simulink model "8Bit_Processor"  (R2019b)
settings: Solver=FixedStepDiscrete  StartTime=0.0  StopTime=10.0  RelTol=1e-3
libraries: hdlsllib x127, simulink_extras x9
(part 1 of 4)
settings Model: Creator=cohen  LastModifiedBy=cohen

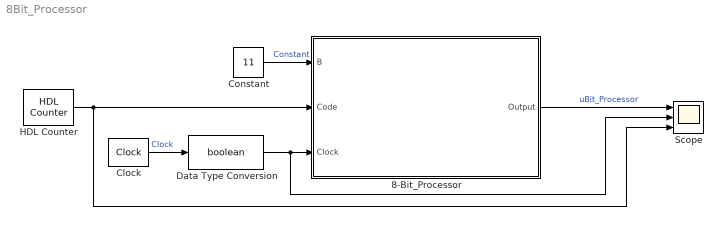
== system 8Bit_Processor ==
  8-Bit_Processor : Subsystem
  Clock : simulink_extras/Flip Flops/Clock  period=1
  Constant : Constant  Value=11  OutDataTypeStr=uint8  SampleTime=1
  Data Type Conversion : DataTypeConversion  OutDataTypeStr=boolean
  HDL Counter : hdlsllib/Sources/HDL Counter  CountType=Free running  CountInit=0  CountStep=1  CountMax=25  CountFromType=Initial value  CountFrom=0  CountResetPort=off  CountLoadPort=off  CountEnbPort=off  CountDirPort=off  CountDataType=Unsigned  CountWordLen=2  CountFracLen=0  CountSampTime=1
      settings: SourceProductName=Simulink
  Scope : Scope  NumInputPorts=3
  wires:
  Constant/1 -> 8-Bit_Processor/1(B)  "Constant"
  Clock/1 -> Data Type Conversion/1  "Clock"
  Data Type Conversion/1 -> Scope/2, 8-Bit_Processor/3(Clock)
  HDL Counter/1 -> Scope/3, 8-Bit_Processor/2(Code)
  8-Bit_Processor/1(Output) -> Scope/1  "uBit_Processor"

== system 8Bit_Processor/8-Bit_Processor ==
  B : Inport  OutDataTypeStr=uint8
  Code : Inport  Port=2
  Clock : Inport  Port=3
  8-Bit 4-to-1 MUX : Subsystem
  8-Bit_Adder : Subsystem
  8-Bit_Bitwise_AND : Subsystem
  8-Bit_Multiplier : Subsystem
  8-Bit_Register : Subsystem
  8-Bit_Subtractor : Subsystem
  Display : Display
  Display1 : Display
  Output : Outport  OutDataTypeStr=uint8
  wires:
  Code/1 -> 8-Bit 4-to-1 MUX/5(S)
  8-Bit 4-to-1 MUX/1(Out1) -> Output/1, Display/1, 8-Bit_Register/1(Data_In)
  Clock/1 -> 8-Bit_Register/2(Clk)
  8-Bit_Multiplier/1(Product) -> 8-Bit 4-to-1 MUX/2(In2)
  8-Bit_Bitwise_AND/1(Y) -> 8-Bit 4-to-1 MUX/4(In4)
  B/1 -> 8-Bit_Multiplier/2(B), 8-Bit_Subtractor/2(B), 8-Bit_Bitwise_AND/2(B), 8-Bit_Adder/2(B)
  8-Bit_Adder/1(Sum) -> 8-Bit 4-to-1 MUX/1(In1)
  8-Bit_Register/1(Data_out) -> Display1/1, 8-Bit_Adder/1(A), 8-Bit_Multiplier/1(A), 8-Bit_Subtractor/1(A), 8-Bit_Bitwise_AND/1(A)
  8-Bit_Subtractor/1(Difference) -> 8-Bit 4-to-1 MUX/3(In3)

== system 8Bit_Processor/8-Bit_Processor/8-Bit 4-to-1 MUX ==
  In1 : Inport  OutDataTypeStr=uint8
  In2 : Inport  Port=2  OutDataTypeStr=uint8
  In3 : Inport  Port=3  OutDataTypeStr=uint8
  In4 : Inport  Port=4  OutDataTypeStr=uint8
  S : Inport  Port=5
  Concat : Subsystem
  Slicer : Subsystem
  Slicer1 : Subsystem
  Slicer2 : Subsystem
  Slicer3 : Subsystem
  Subsystem : Subsystem
  Subsystem1 : Subsystem
  Subsystem2 : Subsystem
  Subsystem3 : Subsystem
  Subsystem4 : Subsystem
  Subsystem5 : Subsystem
  Subsystem6 : Subsystem
  Subsystem7 : Subsystem
  Out1 : Outport  OutDataTypeStr=uint8
  wires:
  Slicer1/8(Y0) -> Subsystem/2(I1)
  Subsystem3/1(Out1) -> Concat/5(X3)
  Slicer/6(Y2) -> Subsystem2/1(I0)
  Slicer2/7(Y1) -> Subsystem1/3(I2)
  Subsystem2/1(Out1) -> Concat/6(X2)
  Concat/1(Y) -> Out1/1
  S/1 -> Subsystem7/5(S), Subsystem4/5(S), Subsystem1/5(S), Subsystem/5(S), Subsystem2/5(S), Subsystem3/5(S), Subsystem5/5(S), Subsystem6/5(S)
  Subsystem6/1(Out1) -> Concat/2(X6)
  Slicer2/3(Y5) -> Subsystem5/3(I2)
  Slicer3/4(Y4) -> Subsystem4/4(I3)
  Slicer2/2(Y6) -> Subsystem6/3(I2)
  Slicer/2(Y6) -> Subsystem6/1(I0)
  In2/1 -> Slicer1/1(X)
  Slicer2/1(Y7) -> Subsystem7/3(I2)
  Slicer3/7(Y1) -> Subsystem1/4(I3)
  Slicer/5(Y3) -> Subsystem3/1(I0)
  Slicer3/6(Y2) -> Subsystem2/4(I3)
  In1/1 -> Slicer/1(X)
  Slicer1/1(Y7) -> Subsystem7/2(I1)
  In3/1 -> Slicer2/1(X)
  Slicer/8(Y0) -> Subsystem/1(I0)
  Slicer1/4(Y4) -> Subsystem4/2(I1)
  Slicer2/4(Y4) -> Subsystem4/3(I2)
  Slicer1/3(Y5) -> Subsystem5/2(I1)
  Slicer3/5(Y3) -> Subsystem3/4(I3)
  Slicer/4(Y4) -> Subsystem4/1(I0)
  Slicer2/8(Y0) -> Subsystem/3(I2)
  Slicer1/5(Y3) -> Subsystem3/2(I1)
  Slicer1/7(Y1) -> Subsystem1/2(I1)
  Subsystem7/1(Out1) -> Concat/1(X7)
  Slicer1/6(Y2) -> Subsystem2/2(I1)
  Subsystem/1(Out1) -> Concat/8(X0)
  Subsystem4/1(Out1) -> Concat/4(X4)
  Subsystem5/1(Out1) -> Concat/3(X5)
  Slicer1/2(Y6) -> Subsystem6/2(I1)
  Slicer3/8(Y0) -> Subsystem/4(I3)
  Slicer2/6(Y2) -> Subsystem2/3(I2)
  Slicer/3(Y5) -> Subsystem5/1(I0)
  Slicer3/3(Y5) -> Subsystem5/4(I3)
  Slicer3/2(Y6) -> Subsystem6/4(I3)
  Slicer3/1(Y7) -> Subsystem7/4(I3)
  Slicer2/5(Y3) -> Subsystem3/3(I2)
  In4/1 -> Slicer3/1(X)
  Subsystem1/1(Out1) -> Concat/7(X1)
  Slicer/1(Y7) -> Subsystem7/1(I0)
  Slicer/7(Y1) -> Subsystem1/1(I0)

== system 8Bit_Processor/8-Bit_Processor/8-Bit_Adder ==
  A : Inport  OutDataTypeStr=uint8
  B : Inport  Port=2  OutDataTypeStr=uint8
  Concat1 : Subsystem
  Full adder1 : Subsystem
  Full adder2 : Subsystem
  Full adder3 : Subsystem
  Full adder4 : Subsystem
  Full adder5 : Subsystem
  Full adder6 : Subsystem
  Full adder7 : Subsystem
  Half adder1 : Subsystem
  Slicer1 : Subsystem
  Slicer2 : Subsystem
  Terminator : Terminator
  Sum : Outport
  wires:
  Slicer1/7(Y1) -> Full adder1/1(In1)
  Full adder2/2(Out2) -> Full adder3/3(In3)
  Slicer1/1(Y7) -> Full adder7/1(In1)
  Full adder5/2(Out2) -> Full adder6/3(In3)
  Slicer1/4(Y4) -> Full adder4/1(In1)
  A/1 -> Slicer1/1(X)
  Slicer1/2(Y6) -> Full adder6/1(In1)
  Full adder6/2(Out2) -> Full adder7/3(In3)
  Full adder6/1(Out1) -> Concat1/2(X6)
  Slicer2/4(Y4) -> Full adder4/2(In2)
  Slicer1/3(Y5) -> Full adder5/1(In1)
  Concat1/1(Y) -> Sum/1
  Full adder3/2(Out2) -> Full adder4/3(In3)
  Full adder4/2(Out2) -> Full adder5/3(In3)
  Full adder1/2(Out2) -> Full adder2/3(In3)
  Slicer2/2(Y6) -> Full adder6/2(In2)
  Slicer1/8(Y0) -> Half adder1/1(In1)
  Slicer2/3(Y5) -> Full adder5/2(In2)
  Slicer2/1(Y7) -> Full adder7/2(In2)
  Full adder3/1(Out1) -> Concat1/5(X3)
  Slicer1/6(Y2) -> Full adder2/1(In1)
  Half adder1/2(Out2) -> Full adder1/3(In3)
  Half adder1/1(Out1) -> Concat1/8(X0)
  Full adder2/1(Out1) -> Concat1/6(X2)
  Slicer2/5(Y3) -> Full adder3/2(In2)
  B/1 -> Slicer2/1(X)
  Full adder7/1(Out1) -> Concat1/1(X7)
  Full adder5/1(Out1) -> Concat1/3(X5)
  Full adder1/1(Out1) -> Concat1/7(X1)
  Full adder4/1(Out1) -> Concat1/4(X4)
  Slicer2/8(Y0) -> Half adder1/2(In2)
  Slicer2/7(Y1) -> Full adder1/2(In2)
  Slicer1/5(Y3) -> Full adder3/1(In1)
  Slicer2/6(Y2) -> Full adder2/2(In2)
  Full adder7/2(Out2) -> Terminator/1

== system 8Bit_Processor/8-Bit_Processor/8-Bit_Bitwise_AND ==
  A : Inport
  B : Inport  Port=2
  Bit Concat : hdlsllib/Logic and Bit Operations/Bit Concat  numInputs=8
      settings: SourceProductName=Simulink
  SliceB : Subsystem
  X0Y0 : Logic  AllPortsSameDT=off  OutDataTypeStr=boolean
  X1Y1 : Logic  AllPortsSameDT=off  OutDataTypeStr=boolean
  X2Y2 : Logic  AllPortsSameDT=off  OutDataTypeStr=boolean
  X3Y3 : Logic  AllPortsSameDT=off  OutDataTypeStr=boolean
  X4Y4 : Logic  AllPortsSameDT=off  OutDataTypeStr=boolean
  X5Y5 : Logic  AllPortsSameDT=off  OutDataTypeStr=boolean
  X6Y6 : Logic  AllPortsSameDT=off  OutDataTypeStr=boolean
  X7Y7 : Logic  AllPortsSameDT=off  OutDataTypeStr=boolean
  sliceA : Subsystem
  Y : Outport
  wires:
  X5Y5/1 -> Bit Concat/3
  B/1 -> SliceB/1(X)
  X3Y3/1 -> Bit Concat/5
  X2Y2/1 -> Bit Concat/6
  A/1 -> sliceA/1(X)
  X6Y6/1 -> Bit Concat/2
  X7Y7/1 -> Bit Concat/1
  X1Y1/1 -> Bit Concat/7
  X0Y0/1 -> Bit Concat/8
  sliceA/6(Y2) -> X2Y2/1
  SliceB/4(Y4) -> X4Y4/2
  X4Y4/1 -> Bit Concat/4
  SliceB/7(Y1) -> X1Y1/2
  sliceA/1(Y7) -> X7Y7/1
  sliceA/3(Y5) -> X5Y5/1
  sliceA/2(Y6) -> X6Y6/1
  sliceA/7(Y1) -> X1Y1/1
  SliceB/6(Y2) -> X2Y2/2
  sliceA/8(Y0) -> X0Y0/1
  SliceB/2(Y6) -> X6Y6/2
  SliceB/3(Y5) -> X5Y5/2
  SliceB/5(Y3) -> X3Y3/2
  sliceA/4(Y4) -> X4Y4/1
  sliceA/5(Y3) -> X3Y3/1
  SliceB/1(Y7) -> X7Y7/2
  SliceB/8(Y0) -> X0Y0/2
  Bit Concat/1 -> Y/1

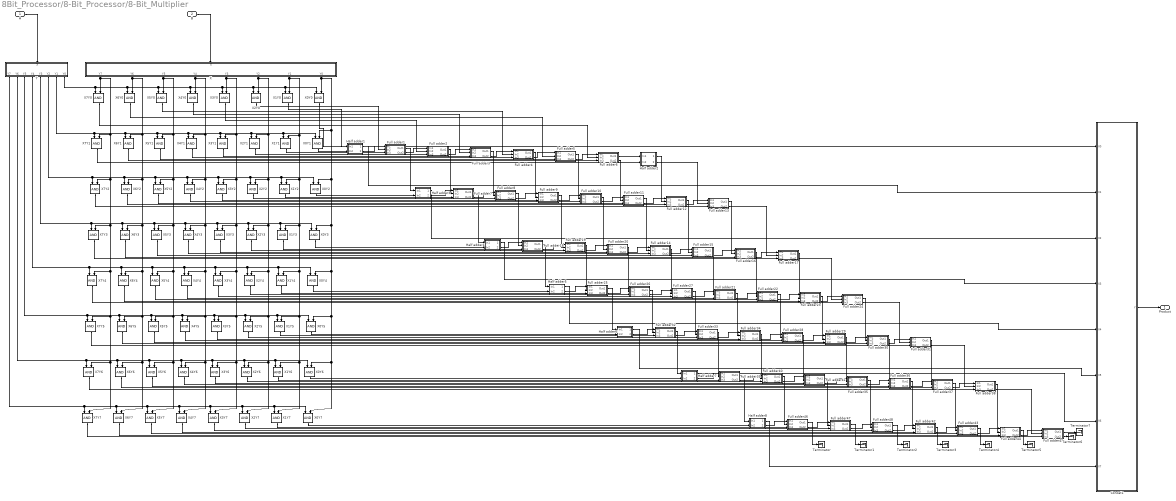
== system 8Bit_Processor/8-Bit_Processor/8-Bit_Multiplier ==
  A : Inport
  B : Inport  Port=2
  Concat1 : Subsystem
  Full adder1 : Subsystem
  Full adder10 : Subsystem
  Full adder11 : Subsystem
  Full adder12 : Subsystem
  Full adder13 : Subsystem
  Full adder14 : Subsystem
  Full adder15 : Subsystem
  Full adder16 : Subsystem
  Full adder17 : Subsystem
  Full adder18 : Subsystem
  Full adder19 : Subsystem
  Full adder2 : Subsystem
  Full adder20 : Subsystem
  Full adder21 : Subsystem
  Full adder22 : Subsystem
  Full adder23 : Subsystem
  Full adder24 : Subsystem
  Full adder25 : Subsystem
  Full adder26 : Subsystem
  Full adder27 : Subsystem
  Full adder28 : Subsystem
  Full adder29 : Subsystem
  Full adder3 : Subsystem
  Full adder30 : Subsystem
  Full adder31 : Subsystem
  Full adder32 : Subsystem
  Full adder33 : Subsystem
  Full adder34 : Subsystem
  Full adder35 : Subsystem
  Full adder36 : Subsystem
  Full adder37 : Subsystem
  Full adder38 : Subsystem
  Full adder39 : Subsystem
  Full adder4 : Subsystem
  Full adder40 : Subsystem
  Full adder41 : Subsystem
  Full adder42 : Subsystem
  Full adder43 : Subsystem
  Full adder44 : Subsystem
  Full adder45 : Subsystem
  Full adder46 : Subsystem
  Full adder47 : Subsystem
  Full adder48 : Subsystem
  Full adder5 : Subsystem
  Full adder6 : Subsystem
  Full adder7 : Subsystem
  Full adder8 : Subsystem
  Full adder9 : Subsystem
  Half adder1 : Subsystem
  Half adder2 : Subsystem
  Half adder3 : Subsystem
  Half adder4 : Subsystem
  Half adder5 : Subsystem
  Half adder6 : Subsystem
  Half adder7 : Subsystem
  Half adder8 : Subsystem
  Terminator{,1..7} (8 alike) : Terminator
  X : Subsystem
  X0Y{0..7} (8 alike) : Logic  AllPortsSameDT=off  OutDataTypeStr=boolean
  X1Y{0..7} (8 alike) : Logic  AllPortsSameDT=off  OutDataTypeStr=boolean
  X2Y{0..7} (8 alike) : Logic  AllPortsSameDT=off  OutDataTypeStr=boolean
  X3Y{0..7} (8 alike) : Logic  AllPortsSameDT=off  OutDataTypeStr=boolean
  X4Y{0..7} (8 alike) : Logic  AllPortsSameDT=off  OutDataTypeStr=boolean
  X5Y{0..7} (8 alike) : Logic  AllPortsSameDT=off  OutDataTypeStr=boolean
  X6Y{0..7} (8 alike) : Logic  AllPortsSameDT=off  OutDataTypeStr=boolean
  X7Y{0..7} (8 alike) : Logic  AllPortsSameDT=off  OutDataTypeStr=boolean
  Y : Subsystem
  Product : Outport
  wires:
  X/3(Y5) -> X5Y1/2, X5Y7/2, X5Y6/2, X5Y5/2, X5Y4/2, X5Y3/2, X5Y2/2, X5Y0/2
  Full adder31/2(Out2) -> Full adder38/2(In2)
  Half adder5/1(Out1) -> Concat1/5(X4)
  Full adder4/1(Out1) -> Full adder9/2(In2)
  Full adder15/1(Out1) -> Full adder21/2(In2)
  Full adder10/2(Out2) -> Full adder11/1(In1)
  Full adder3/2(Out2) -> Full adder4/1(In1)
  Full adder7/2(Out2) -> Full adder8/1(In1)
  X/8(Y0) -> X0Y7/2, X0Y6/2, X0Y5/2, X0Y4/2, X0Y3/2, X0Y2/2, X0Y1/2, X0Y0/2
  Full adder21/2(Out2) -> Full adder22/1(In1)
  Full adder5/1(Out1) -> Full adder10/2(In2)
  X/4(Y4) -> X4Y1/2, X4Y7/2, X4Y6/2, X4Y5/2, X4Y4/2, X4Y3/2, X4Y2/2, X4Y0/2
  X6Y4/1 -> Full adder23/3(In3)
  Full adder11/2(Out2) -> Full adder12/1(In1)
  X/5(Y3) -> X3Y1/2, X3Y7/2, X3Y6/2, X3Y5/2, X3Y4/2, X3Y3/2, X3Y2/2, X3Y0/2
  Full adder15/2(Out2) -> Full adder16/1(In1)
  Full adder32/1(Out1) -> Half adder7/1(In1)
  X5Y6/1 -> Full adder36/3(In3)
  Full adder38/2(Out2) -> Full adder45/2(In2)
  Full adder46/2(Out2) -> Full adder47/1(In1)
  Full adder6/2(Out2) -> Full adder11/2(In2)
  X5Y5/1 -> Full adder29/3(In3)
  X/2(Y6) -> X6Y1/2, X6Y7/2, X6Y6/2, X6Y5/2, X6Y4/2, X6Y3/2, X6Y2/2, X6Y0/2
  Full adder44/2(Out2) -> Full adder45/1(In1)
  Half adder4/1(Out1) -> Concat1/4(X3)
  Full adder38/1(Out1) -> Full adder44/2(In2)
  X/1(Y7) -> X7Y1/2, X7Y7/2, X7Y6/2, X7Y5/2, X7Y4/2, X7Y3/2, X7Y2/2, X7Y0/2
  Full adder8/2(Out2) -> Full adder9/1(In1)
  Full adder43/2(Out2) -> Full adder44/1(In1)
  Y/7(Y1) -> X7Y1/1, X6Y1/1, X5Y1/1, X4Y1/1, X3Y1/1, X2Y1/1, X1Y1/1, X0Y1/1
  X/6(Y2) -> X2Y1/2, X2Y7/2, X2Y6/2, X2Y5/2, X2Y4/2, X2Y3/2, X2Y2/2, X2Y0/2
  Half adder8/2(Out2) -> Full adder46/1(In1)
  Full adder13/2(Out2) -> Full adder17/2(In2)
  X1Y1/1 -> Full adder1/3(In3)
  Half adder6/1(Out1) -> Concat1/6(X5)
  Half adder3/2(Out2) -> Full adder7/1(In1)
  X4Y6/1 -> Full adder35/3(In3)
  Full adder11/1(Out1) -> Full adder14/2(In2)
  Full adder27/1(Out1) -> Full adder33/2(In2)
  Full adder42/2(Out2) -> Full adder43/1(In1)
  Y/4(Y4) -> X7Y4/1, X6Y4/1, X5Y4/1, X4Y4/1, X3Y4/1, X2Y4/1, X1Y4/1, X0Y4/1
  Full adder33/2(Out2) -> Full adder34/1(In1)
  Full adder23/1(Out1) -> Full adder29/2(In2)
  X0Y0/1 -> Concat1/1(X0)
  Full adder18/2(Out2) -> Full adder19/1(In1)
  Full adder37/2(Out2) -> Full adder38/1(In1)
  Full adder36/1(Out1) -> Full adder42/2(In2)
  Full adder37/1(Out1) -> Full adder43/2(In2)
  Y/3(Y5) -> X7Y5/1, X6Y5/1, X5Y5/1, X4Y5/1, X3Y5/1, X2Y5/1, X1Y5/1, X0Y5/1
  Half adder3/1(Out1) -> Concat1/3(X2)
  Half adder4/2(Out2) -> Full adder18/1(In1)
  X2Y2/1 -> Full adder8/3(In3)
  X7Y1/1 -> Half adder2/2(In2)
  Full adder17/2(Out2) -> Full adder24/2(In2)
  Y/2(Y6) -> X7Y6/1, X6Y6/1, X5Y6/1, X4Y6/1, X3Y6/1, X2Y6/1, X1Y6/1, X0Y6/1
  Half adder6/2(Out2) -> Full adder32/1(In1)
  Full adder23/2(Out2) -> Full adder24/1(In1)
  Full adder21/1(Out1) -> Full adder34/2(In2)
  X/7(Y1) -> X1Y1/2, X1Y7/2, X1Y6/2, X1Y5/2, X1Y4/2, X1Y3/2, X1Y2/2, X1Y0/2
  Y/6(Y2) -> X7Y2/1, X6Y2/1, X5Y2/1, X4Y2/1, X3Y2/1, X1Y2/1, X0Y2/1, X2Y2/1
  Full adder31/1(Out1) -> Full adder37/2(In2)
  Half adder1/1(Out1) -> Concat1/2(X1)
  X5Y4/1 -> Full adder22/3(In3)
  Full adder8/1(Out1) -> Full adder18/2(In2)
  Full adder40/1(Out1) -> Full adder46/2(In2)
  Half adder2/1(Out1) -> Full adder12/2(In2)
  Full adder19/2(Out2) -> Full adder20/1(In1)
  Y/8(Y0) -> X7Y0/1, X6Y0/1, X5Y0/1, X4Y0/1, X3Y0/1, X2Y0/1, X1Y0/1, X0Y0/1
  Full adder1/2(Out2) -> Full adder2/1(In1)
  Full adder16/1(Out1) -> Full adder22/2(In2)
  Full adder28/2(Out2) -> Full adder29/1(In1)
  Full adder12/2(Out2) -> Full adder13/1(In1)
  Full adder12/1(Out1) -> Full adder15/2(In2)
  Full adder10/1(Out1) -> Full adder20/2(In2)
  Y/5(Y3) -> X7Y3/1, X6Y3/1, X5Y3/1, X4Y3/1, X3Y3/1, X2Y3/1, X1Y3/1, X0Y3/1
  Full adder32/2(Out2) -> Full adder33/1(In1)
  Full adder26/1(Out1) -> Full adder32/2(In2)
  X3Y5/1 -> Full adder34/3(In3)
  Half adder8/1(Out1) -> Concat1/8(X7)
  Full adder26/2(Out2) -> Full adder27/1(In1)
  Full adder9/2(Out2) -> Full adder10/1(In1)
  Half adder7/2(Out2) -> Full adder39/1(In1)
  Full adder24/1(Out1) -> Full adder30/2(In2)
  Full adder41/2(Out2) -> Full adder35/1(In1)
  Full adder3/1(Out1) -> Full adder8/2(In2)
  Full adder39/1(Out1) -> Half adder8/1(In1)
  Full adder35/1(Out1) -> Full adder48/2(In2)
  Full adder5/2(Out2) -> Full adder6/1(In1)
  Full adder9/1(Out1) -> Full adder19/2(In2)
  Full adder35/2(Out2) -> Full adder36/1(In1)
  Full adder40/2(Out2) -> Full adder41/1(In1)
  X1Y5/1 -> Full adder32/3(In3)
  X2Y6/1 -> Full adder40/3(In3)
  Full adder48/2(Out2) -> Full adder42/1(In1)
  Full adder27/2(Out2) -> Full adder21/1(In1)
  Full adder47/2(Out2) -> Full adder48/1(In1)
  X7Y5/1 -> Full adder31/3(In3)
  Full adder28/1(Out1) -> Full adder41/2(In2)
  Full adder20/2(Out2) -> Full adder14/1(In1)
  X6Y3/1 -> Full adder16/3(In3)
  Full adder7/1(Out1) -> Half adder4/1(In1)
  Full adder34/1(Out1) -> Full adder40/2(In2)
  Full adder29/1(Out1) -> Full adder35/2(In2)
  Full adder34/2(Out2) -> Full adder28/1(In1)
  Full adder22/2(Out2) -> Full adder23/1(In1)
  X6Y5/1 -> Full adder30/3(In3)
  Full adder41/1(Out1) -> Full adder47/2(In2)
  Half adder5/2(Out2) -> Full adder25/1(In1)
  B/1 -> X/1(X)
  X1Y3/1 -> Full adder18/3(In3)
  X4Y3/1 -> Full adder14/3(In3)
  Full adder2/2(Out2) -> Full adder3/1(In1)
  Full adder13/1(Out1) -> Full adder16/2(In2)
  Full adder25/2(Out2) -> Full adder26/1(In1)
  X3Y0/1 -> Full adder2/2(In2)
  Full adder33/1(Out1) -> Full adder39/2(In2)
  Full adder18/1(Out1) -> Half adder5/1(In1)
  Full adder29/2(Out2) -> Full adder30/1(In1)
  X5Y1/1 -> Full adder5/3(In3)
  A/1 -> Y/1(X)
  X2Y5/1 -> Full adder33/3(In3)
  Full adder25/1(Out1) -> Half adder6/1(In1)
  X4Y4/1 -> Full adder21/3(In3)
  Full adder30/1(Out1) -> Full adder36/2(In2)
  Full adder24/2(Out2) -> Full adder31/2(In2)
  Concat1/1(Y) -> Product/1
  Full adder39/2(Out2) -> Full adder40/1(In1)
  Full adder36/2(Out2) -> Full adder37/1(In1)
  Half adder2/2(Out2) -> Full adder13/2(In2)
  Half adder7/1(Out1) -> Concat1/7(X6)
  Full adder16/2(Out2) -> Full adder17/1(In1)
  X0Y4/1 -> Half adder5/2(In2)
  Full adder20/1(Out1) -> Full adder26/2(In2)
  X5Y3/1 -> Full adder15/3(In3)
  X2Y0/1 -> Full adder1/2(In2)
  Half adder1/2(Out2) -> Full adder1/1(In1)
  Full adder22/1(Out1) -> Full adder28/2(In2)
  X2Y3/1 -> Full adder19/3(In3)
  Full adder4/2(Out2) -> Full adder5/1(In1)
  X6Y1/1 -> Full adder6/3(In3)
  Full adder14/2(Out2) -> Full adder15/1(In1)
  Full adder1/1(Out1) -> Half adder3/1(In1)
  Full adder2/1(Out1) -> Full adder7/2(In2)
  Full adder30/2(Out2) -> Full adder31/1(In1)
  Full adder14/1(Out1) -> Full adder27/2(In2)
  X7Y7/1 -> Full adder45/3(In3)
  Full adder17/1(Out1) -> Full adder23/2(In2)
  Y/1(Y7) -> X7Y7/1, X6Y7/1, X5Y7/1, X4Y7/1, X3Y7/1, X2Y7/1, X1Y7/1, X0Y7/1
  Full adder19/1(Out1) -> Full adder25/2(In2)
  X2Y7/1 -> Full adder47/3(In3)
  X2Y4/1 -> Full adder26/3(In3)
  X0Y1/1 -> Half adder1/2(In2)
  X5Y7/1 -> Full adder43/3(In3)
  X5Y2/1 -> Full adder11/3(In3)
  X1Y2/1 -> Full adder7/3(In3)
  X1Y0/1 -> Half adder1/1(In1)
  X0Y3/1 -> Half adder4/2(In2)
  X4Y1/1 -> Full adder4/3(In3)
  X1Y7/1 -> Full adder46/3(In3)
  X7Y4/1 -> Full adder24/3(In3)
  X4Y0/1 -> Full adder3/2(In2)
  X3Y1/1 -> Full adder3/3(In3)
  X3Y3/1 -> Full adder20/3(In3)
  X7Y0/1 -> Full adder6/2(In2)
  X1Y6/1 -> Full adder39/3(In3)
  Full adder6/1(Out1) -> Half adder2/1(In1)
  X5Y0/1 -> Full adder4/2(In2)
  X6Y7/1 -> Full adder44/3(In3)
  X1Y4/1 -> Full adder25/3(In3)
  X0Y2/1 -> Half adder3/2(In2)
  X7Y3/1 -> Full adder17/3(In3)
  X4Y2/1 -> Full adder10/3(In3)
  X7Y2/1 -> Full adder13/3(In3)
  X3Y2/1 -> Full adder9/3(In3)
  X6Y2/1 -> Full adder12/3(In3)
  X3Y4/1 -> Full adder27/3(In3)
  X7Y6/1 -> Full adder38/3(In3)
  X0Y5/1 -> Half adder6/2(In2)
  X4Y5/1 -> Full adder28/3(In3)
  X6Y0/1 -> Full adder5/2(In2)
  X0Y6/1 -> Half adder7/2(In2)
  X4Y7/1 -> Full adder42/3(In3)
  X2Y1/1 -> Full adder2/3(In3)
  X3Y7/1 -> Full adder48/3(In3)
  X6Y6/1 -> Full adder37/3(In3)
  X0Y7/1 -> Half adder8/2(In2)
  X3Y6/1 -> Full adder41/3(In3)
  Full adder46/1(Out1) -> Terminator/1
  Full adder47/1(Out1) -> Terminator1/1
  Full adder48/1(Out1) -> Terminator2/1
  Full adder42/1(Out1) -> Terminator3/1
  Full adder43/1(Out1) -> Terminator4/1
  Full adder44/1(Out1) -> Terminator5/1
  Full adder45/2(Out2) -> Terminator6/1
  Full adder45/1(Out1) -> Terminator7/1

== system 8Bit_Processor/8-Bit_Processor/8-Bit_Register ==
  Data_In : Inport  OutDataTypeStr=uint8
  Clk : Inport  Port=2
  Concat : Subsystem
  Constant : Constant  OutDataTypeStr=boolean  SampleTime=1
  D Flip-Flop{,1..7} (8 alike) : simulink_extras/Flip Flops/D Flip-Flop
      settings: SourceProductName=Simulink
  Slicer : Subsystem
  Terminator{,1..7} (8 alike) : Terminator
  Data_out : Outport  OutDataTypeStr=uint8
  wires:
  D Flip-Flop6/1 -> Concat/7(X6)
  Slicer/3(Y5) -> D Flip-Flop5/1
  D Flip-Flop5/1 -> Concat/6(X5)
  D Flip-Flop2/1 -> Concat/3(X2)
  Constant/1 -> D Flip-Flop/3, D Flip-Flop2/3, D Flip-Flop3/3, D Flip-Flop4/3, D Flip-Flop5/3, D Flip-Flop6/3, D Flip-Flop7/3, D Flip-Flop1/3
  Clk/1 -> D Flip-Flop/2, D Flip-Flop1/2, D Flip-Flop2/2, D Flip-Flop3/2, D Flip-Flop4/2, D Flip-Flop6/2, D Flip-Flop7/2, D Flip-Flop5/2
  D Flip-Flop4/1 -> Concat/5(X4)
  D Flip-Flop2/2 -> Terminator2/1
  Slicer/5(Y3) -> D Flip-Flop3/1
  Slicer/1(Y7) -> D Flip-Flop7/1
  Concat/1(Y) -> Data_out/1
  D Flip-Flop5/2 -> Terminator5/1
  D Flip-Flop7/1 -> Concat/8(X7)
  Slicer/7(Y1) -> D Flip-Flop1/1
  D Flip-Flop1/1 -> Concat/2(X1)
  D Flip-Flop6/2 -> Terminator6/1
  Slicer/6(Y2) -> D Flip-Flop2/1
  D Flip-Flop3/1 -> Concat/4(X3)
  D Flip-Flop/1 -> Concat/1(X0)
  D Flip-Flop4/2 -> Terminator4/1
  D Flip-Flop3/2 -> Terminator3/1
  D Flip-Flop7/2 -> Terminator7/1
  D Flip-Flop/2 -> Terminator/1
  Slicer/4(Y4) -> D Flip-Flop4/1
  Data_In/1 -> Slicer/1(X)
  Slicer/8(Y0) -> D Flip-Flop/1
  Slicer/2(Y6) -> D Flip-Flop6/1
  D Flip-Flop1/2 -> Terminator1/1

== system 8Bit_Processor/8-Bit_Processor/8-Bit_Subtractor ==
  A : Inport  OutDataTypeStr=uint8
  B : Inport  Port=2  OutDataTypeStr=uint8
  Concat1 : Subsystem
  Full Subtractor : Subsystem
  Full Subtractor 2 : Subsystem
  Full Subtractor 3 : Subsystem
  Full Subtractor 4 : Subsystem
  Full Subtractor 5 : Subsystem
  Full Subtractor 6 : Subsystem
  Full Subtractor 7 : Subsystem
  Half subtractor : Subsystem
  Slicer1 : Subsystem
  Slicer2 : Subsystem
  Terminator : Terminator
  Difference : Outport
  wires:
  Slicer1/7(Y1) -> Full Subtractor/1(In1)
  Full Subtractor 2/2(Out2) -> Full Subtractor 3/3(In3)
  Slicer1/1(Y7) -> Full Subtractor 7/1(In1)
  Full Subtractor 5/2(Out2) -> Full Subtractor 6/3(In3)
  Slicer1/4(Y4) -> Full Subtractor 4/1(In1)
  A/1 -> Slicer1/1(X)
  Slicer1/2(Y6) -> Full Subtractor 6/1(In1)
  Full Subtractor 6/2(Out2) -> Full Subtractor 7/3(In3)
  Full Subtractor 6/1(Out1) -> Concat1/2(X6)
  Slicer2/4(Y4) -> Full Subtractor 4/2(In2)
  Slicer1/3(Y5) -> Full Subtractor 5/1(In1)
  Concat1/1(Y) -> Difference/1
  Full Subtractor 3/2(Out2) -> Full Subtractor 4/3(In3)
  Full Subtractor 4/2(Out2) -> Full Subtractor 5/3(In3)
  Full Subtractor/2(Out2) -> Full Subtractor 2/3(In3)
  Slicer2/2(Y6) -> Full Subtractor 6/2(In2)
  Slicer1/8(Y0) -> Half subtractor/1(In1)
  Slicer2/3(Y5) -> Full Subtractor 5/2(In2)
  Slicer2/1(Y7) -> Full Subtractor 7/2(In2)
  Full Subtractor 3/1(Out1) -> Concat1/5(X3)
  Slicer1/6(Y2) -> Full Subtractor 2/1(In1)
  Half subtractor/2(Out2) -> Full Subtractor/3(In3)
  Half subtractor/1(Out1) -> Concat1/8(X0)
  Full Subtractor 2/1(Out1) -> Concat1/6(X2)
  Slicer2/5(Y3) -> Full Subtractor 3/2(In2)
  B/1 -> Slicer2/1(X)
  Full Subtractor 7/1(Out1) -> Concat1/1(X7)
  Full Subtractor 5/1(Out1) -> Concat1/3(X5)
  Full Subtractor/1(Out1) -> Concat1/7(X1)
  Full Subtractor 4/1(Out1) -> Concat1/4(X4)
  Slicer2/8(Y0) -> Half subtractor/2(In2)
  Slicer2/7(Y1) -> Full Subtractor/2(In2)
  Slicer1/5(Y3) -> Full Subtractor 3/1(In1)
  Slicer2/6(Y2) -> Full Subtractor 2/2(In2)
  Full Subtractor 7/2(Out2) -> Terminator/1

== system 8Bit_Processor/8-Bit_Processor/8-Bit 4-to-1 MUX/Concat ==
  X7 : Inport  OutDataTypeStr=boolean  SampleTime=1
  X6 : Inport  Port=2  OutDataTypeStr=boolean  SampleTime=1
  X5 : Inport  Port=3  OutDataTypeStr=boolean  SampleTime=1
  X4 : Inport  Port=4  OutDataTypeStr=boolean  SampleTime=1
  X3 : Inport  Port=5  OutDataTypeStr=boolean  SampleTime=1
  X2 : Inport  Port=6  OutDataTypeStr=boolean  SampleTime=1
  X1 : Inport  Port=7  OutDataTypeStr=boolean  SampleTime=1
  X0 : Inport  Port=8  OutDataTypeStr=boolean  SampleTime=1
  Bit Concat : hdlsllib/Logic and Bit Operations/Bit Concat  numInputs=8
      settings: SourceProductName=Simulink
  Y : Outport  OutDataTypeStr=uint8  SampleTime=1
  wires:
  X6/1 -> Bit Concat/2
  X2/1 -> Bit Concat/6
  X7/1 -> Bit Concat/1
  X0/1 -> Bit Concat/8
  Bit Concat/1 -> Y/1
  X3/1 -> Bit Concat/5
  X1/1 -> Bit Concat/7
  X5/1 -> Bit Concat/3
  X4/1 -> Bit Concat/4

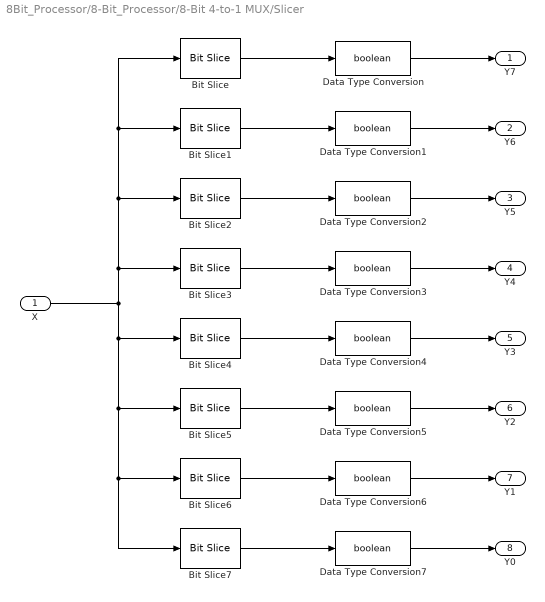
== system 8Bit_Processor/8-Bit_Processor/8-Bit 4-to-1 MUX/Slicer ==
  X : Inport  OutDataTypeStr=uint8  SampleTime=1
  Bit Slice : hdlsllib/Logic and Bit Operations/Bit Slice  lidx=7  ridx=7
      settings: SourceProductName=Simulink  SourceProductBaseCode=SL
  Bit Slice1 : hdlsllib/Logic and Bit Operations/Bit Slice  lidx=6  ridx=6
      settings: SourceProductName=Simulink  SourceProductBaseCode=SL
  Bit Slice2 : hdlsllib/Logic and Bit Operations/Bit Slice  lidx=5  ridx=5
      settings: SourceProductName=Simulink  SourceProductBaseCode=SL
  Bit Slice3 : hdlsllib/Logic and Bit Operations/Bit Slice  lidx=4  ridx=4
      settings: SourceProductName=Simulink  SourceProductBaseCode=SL
  Bit Slice4 : hdlsllib/Logic and Bit Operations/Bit Slice  lidx=3  ridx=3
      settings: SourceProductName=Simulink  SourceProductBaseCode=SL
  Bit Slice5 : hdlsllib/Logic and Bit Operations/Bit Slice  lidx=2  ridx=2
      settings: SourceProductName=Simulink  SourceProductBaseCode=SL
  Bit Slice6 : hdlsllib/Logic and Bit Operations/Bit Slice  lidx=1  ridx=1
      settings: SourceProductName=Simulink  SourceProductBaseCode=SL
  Bit Slice7 : hdlsllib/Logic and Bit Operations/Bit Slice  lidx=0  ridx=0
      settings: SourceProductName=Simulink  SourceProductBaseCode=SL
  Data Type Conversion{,1..7} (8 alike) : DataTypeConversion  OutDataTypeStr=boolean
  Y7 : Outport  OutDataTypeStr=boolean  SampleTime=1
  Y6 : Outport  Port=2  OutDataTypeStr=boolean  SampleTime=1
  Y5 : Outport  Port=3  OutDataTypeStr=boolean  SampleTime=1
  Y4 : Outport  Port=4  OutDataTypeStr=boolean
  Y3 : Outport  Port=5  OutDataTypeStr=boolean  SampleTime=1
  Y2 : Outport  Port=6  OutDataTypeStr=boolean  SampleTime=1
  Y1 : Outport  Port=7  OutDataTypeStr=boolean  SampleTime=1
  Y0 : Outport  Port=8  OutDataTypeStr=boolean  SampleTime=1
  wires:
  Bit Slice6/1 -> Data Type Conversion6/1
  X/1 -> Bit Slice3/1, Bit Slice2/1, Bit Slice1/1, Bit Slice/1, Bit Slice4/1, Bit Slice5/1, Bit Slice6/1, Bit Slice7/1
  Bit Slice/1 -> Data Type Conversion/1
  Bit Slice7/1 -> Data Type Conversion7/1
  Bit Slice4/1 -> Data Type Conversion4/1
  Bit Slice1/1 -> Data Type Conversion1/1
  Bit Slice3/1 -> Data Type Conversion3/1
  Data Type Conversion1/1 -> Y6/1
  Data Type Conversion7/1 -> Y0/1
  Data Type Conversion5/1 -> Y2/1
  Data Type Conversion3/1 -> Y4/1
  Data Type Conversion4/1 -> Y3/1
  Bit Slice2/1 -> Data Type Conversion2/1
  Bit Slice5/1 -> Data Type Conversion5/1
  Data Type Conversion6/1 -> Y1/1
  Data Type Conversion/1 -> Y7/1
  Data Type Conversion2/1 -> Y5/1

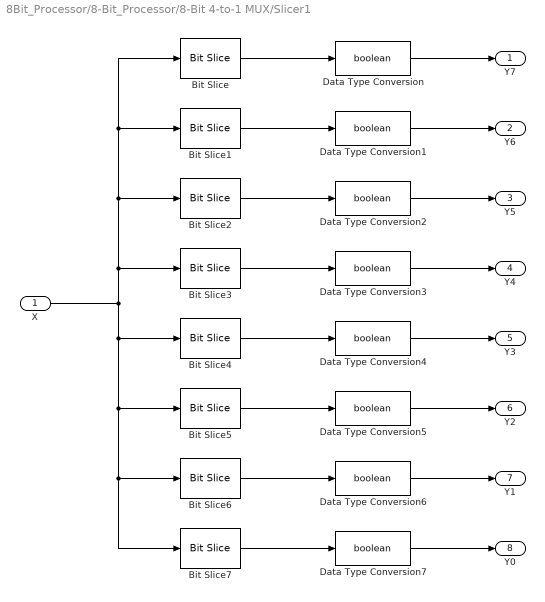
== system 8Bit_Processor/8-Bit_Processor/8-Bit 4-to-1 MUX/Slicer1 ==
  X : Inport  OutDataTypeStr=uint8  SampleTime=1
  Bit Slice : hdlsllib/Logic and Bit Operations/Bit Slice  lidx=7  ridx=7
      settings: SourceProductName=Simulink  SourceProductBaseCode=SL
  Bit Slice1 : hdlsllib/Logic and Bit Operations/Bit Slice  lidx=6  ridx=6
      settings: SourceProductName=Simulink  SourceProductBaseCode=SL
  Bit Slice2 : hdlsllib/Logic and Bit Operations/Bit Slice  lidx=5  ridx=5
      settings: SourceProductName=Simulink  SourceProductBaseCode=SL
  Bit Slice3 : hdlsllib/Logic and Bit Operations/Bit Slice  lidx=4  ridx=4
      settings: SourceProductName=Simulink  SourceProductBaseCode=SL
  Bit Slice4 : hdlsllib/Logic and Bit Operations/Bit Slice  lidx=3  ridx=3
      settings: SourceProductName=Simulink  SourceProductBaseCode=SL
  Bit Slice5 : hdlsllib/Logic and Bit Operations/Bit Slice  lidx=2  ridx=2
      settings: SourceProductName=Simulink  SourceProductBaseCode=SL
  Bit Slice6 : hdlsllib/Logic and Bit Operations/Bit Slice  lidx=1  ridx=1
      settings: SourceProductName=Simulink  SourceProductBaseCode=SL
  Bit Slice7 : hdlsllib/Logic and Bit Operations/Bit Slice  lidx=0  ridx=0
      settings: SourceProductName=Simulink  SourceProductBaseCode=SL
  Data Type Conversion{,1..7} (8 alike) : DataTypeConversion  OutDataTypeStr=boolean
  Y7 : Outport  OutDataTypeStr=boolean  SampleTime=1
  Y6 : Outport  Port=2  OutDataTypeStr=boolean  SampleTime=1
  Y5 : Outport  Port=3  OutDataTypeStr=boolean  SampleTime=1
  Y4 : Outport  Port=4  OutDataTypeStr=boolean
  Y3 : Outport  Port=5  OutDataTypeStr=boolean  SampleTime=1
  Y2 : Outport  Port=6  OutDataTypeStr=boolean  SampleTime=1
  Y1 : Outport  Port=7  OutDataTypeStr=boolean  SampleTime=1
  Y0 : Outport  Port=8  OutDataTypeStr=boolean  SampleTime=1
  wires:
  Bit Slice6/1 -> Data Type Conversion6/1
  X/1 -> Bit Slice3/1, Bit Slice2/1, Bit Slice1/1, Bit Slice/1, Bit Slice4/1, Bit Slice5/1, Bit Slice6/1, Bit Slice7/1
  Bit Slice/1 -> Data Type Conversion/1
  Bit Slice7/1 -> Data Type Conversion7/1
  Bit Slice4/1 -> Data Type Conversion4/1
  Bit Slice1/1 -> Data Type Conversion1/1
  Bit Slice3/1 -> Data Type Conversion3/1
  Data Type Conversion1/1 -> Y6/1
  Data Type Conversion7/1 -> Y0/1
  Data Type Conversion5/1 -> Y2/1
  Data Type Conversion3/1 -> Y4/1
  Data Type Conversion4/1 -> Y3/1
  Bit Slice2/1 -> Data Type Conversion2/1
  Bit Slice5/1 -> Data Type Conversion5/1
  Data Type Conversion6/1 -> Y1/1
  Data Type Conversion/1 -> Y7/1
  Data Type Conversion2/1 -> Y5/1

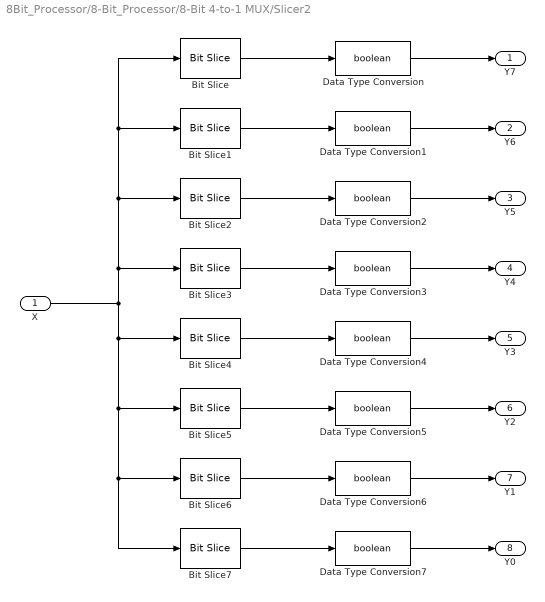
== system 8Bit_Processor/8-Bit_Processor/8-Bit 4-to-1 MUX/Slicer2 ==
  X : Inport  OutDataTypeStr=uint8  SampleTime=1
  Bit Slice : hdlsllib/Logic and Bit Operations/Bit Slice  lidx=7  ridx=7
      settings: SourceProductName=Simulink  SourceProductBaseCode=SL
  Bit Slice1 : hdlsllib/Logic and Bit Operations/Bit Slice  lidx=6  ridx=6
      settings: SourceProductName=Simulink  SourceProductBaseCode=SL
  Bit Slice2 : hdlsllib/Logic and Bit Operations/Bit Slice  lidx=5  ridx=5
      settings: SourceProductName=Simulink  SourceProductBaseCode=SL
  Bit Slice3 : hdlsllib/Logic and Bit Operations/Bit Slice  lidx=4  ridx=4
      settings: SourceProductName=Simulink  SourceProductBaseCode=SL
  Bit Slice4 : hdlsllib/Logic and Bit Operations/Bit Slice  lidx=3  ridx=3
      settings: SourceProductName=Simulink  SourceProductBaseCode=SL
  Bit Slice5 : hdlsllib/Logic and Bit Operations/Bit Slice  lidx=2  ridx=2
      settings: SourceProductName=Simulink  SourceProductBaseCode=SL
  Bit Slice6 : hdlsllib/Logic and Bit Operations/Bit Slice  lidx=1  ridx=1
      settings: SourceProductName=Simulink  SourceProductBaseCode=SL
  Bit Slice7 : hdlsllib/Logic and Bit Operations/Bit Slice  lidx=0  ridx=0
      settings: SourceProductName=Simulink  SourceProductBaseCode=SL
  Data Type Conversion{,1..7} (8 alike) : DataTypeConversion  OutDataTypeStr=boolean
  Y7 : Outport  OutDataTypeStr=boolean  SampleTime=1
  Y6 : Outport  Port=2  OutDataTypeStr=boolean  SampleTime=1
  Y5 : Outport  Port=3  OutDataTypeStr=boolean  SampleTime=1
  Y4 : Outport  Port=4  OutDataTypeStr=boolean
  Y3 : Outport  Port=5  OutDataTypeStr=boolean  SampleTime=1
  Y2 : Outport  Port=6  OutDataTypeStr=boolean  SampleTime=1
  Y1 : Outport  Port=7  OutDataTypeStr=boolean  SampleTime=1
  Y0 : Outport  Port=8  OutDataTypeStr=boolean  SampleTime=1
  wires:
  Bit Slice6/1 -> Data Type Conversion6/1
  X/1 -> Bit Slice3/1, Bit Slice2/1, Bit Slice1/1, Bit Slice/1, Bit Slice4/1, Bit Slice5/1, Bit Slice6/1, Bit Slice7/1
  Bit Slice/1 -> Data Type Conversion/1
  Bit Slice7/1 -> Data Type Conversion7/1
  Bit Slice4/1 -> Data Type Conversion4/1
  Bit Slice1/1 -> Data Type Conversion1/1
  Bit Slice3/1 -> Data Type Conversion3/1
  Data Type Conversion1/1 -> Y6/1
  Data Type Conversion7/1 -> Y0/1
  Data Type Conversion5/1 -> Y2/1
  Data Type Conversion3/1 -> Y4/1
  Data Type Conversion4/1 -> Y3/1
  Bit Slice2/1 -> Data Type Conversion2/1
  Bit Slice5/1 -> Data Type Conversion5/1
  Data Type Conversion6/1 -> Y1/1
  Data Type Conversion/1 -> Y7/1
  Data Type Conversion2/1 -> Y5/1

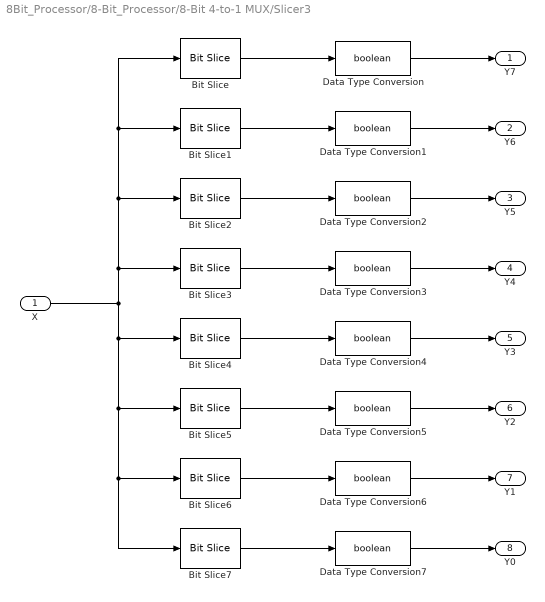
== system 8Bit_Processor/8-Bit_Processor/8-Bit 4-to-1 MUX/Slicer3 ==
  X : Inport  OutDataTypeStr=uint8  SampleTime=1
  Bit Slice : hdlsllib/Logic and Bit Operations/Bit Slice  lidx=7  ridx=7
      settings: SourceProductName=Simulink  SourceProductBaseCode=SL
  Bit Slice1 : hdlsllib/Logic and Bit Operations/Bit Slice  lidx=6  ridx=6
      settings: SourceProductName=Simulink  SourceProductBaseCode=SL
  Bit Slice2 : hdlsllib/Logic and Bit Operations/Bit Slice  lidx=5  ridx=5
      settings: SourceProductName=Simulink  SourceProductBaseCode=SL
  Bit Slice3 : hdlsllib/Logic and Bit Operations/Bit Slice  lidx=4  ridx=4
      settings: SourceProductName=Simulink  SourceProductBaseCode=SL
  Bit Slice4 : hdlsllib/Logic and Bit Operations/Bit Slice  lidx=3  ridx=3
      settings: SourceProductName=Simulink  SourceProductBaseCode=SL
  Bit Slice5 : hdlsllib/Logic and Bit Operations/Bit Slice  lidx=2  ridx=2
      settings: SourceProductName=Simulink  SourceProductBaseCode=SL
  Bit Slice6 : hdlsllib/Logic and Bit Operations/Bit Slice  lidx=1  ridx=1
      settings: SourceProductName=Simulink  SourceProductBaseCode=SL
  Bit Slice7 : hdlsllib/Logic and Bit Operations/Bit Slice  lidx=0  ridx=0
      settings: SourceProductName=Simulink  SourceProductBaseCode=SL
  Data Type Conversion{,1..7} (8 alike) : DataTypeConversion  OutDataTypeStr=boolean
  Y7 : Outport  OutDataTypeStr=boolean  SampleTime=1
  Y6 : Outport  Port=2  OutDataTypeStr=boolean  SampleTime=1
  Y5 : Outport  Port=3  OutDataTypeStr=boolean  SampleTime=1
  Y4 : Outport  Port=4  OutDataTypeStr=boolean
  Y3 : Outport  Port=5  OutDataTypeStr=boolean  SampleTime=1
  Y2 : Outport  Port=6  OutDataTypeStr=boolean  SampleTime=1
  Y1 : Outport  Port=7  OutDataTypeStr=boolean  SampleTime=1
  Y0 : Outport  Port=8  OutDataTypeStr=boolean  SampleTime=1
  wires:
  Bit Slice6/1 -> Data Type Conversion6/1
  X/1 -> Bit Slice3/1, Bit Slice2/1, Bit Slice1/1, Bit Slice/1, Bit Slice4/1, Bit Slice5/1, Bit Slice6/1, Bit Slice7/1
  Bit Slice/1 -> Data Type Conversion/1
  Bit Slice7/1 -> Data Type Conversion7/1
  Bit Slice4/1 -> Data Type Conversion4/1
  Bit Slice1/1 -> Data Type Conversion1/1
  Bit Slice3/1 -> Data Type Conversion3/1
  Data Type Conversion1/1 -> Y6/1
  Data Type Conversion7/1 -> Y0/1
  Data Type Conversion5/1 -> Y2/1
  Data Type Conversion3/1 -> Y4/1
  Data Type Conversion4/1 -> Y3/1
  Bit Slice2/1 -> Data Type Conversion2/1
  Bit Slice5/1 -> Data Type Conversion5/1
  Data Type Conversion6/1 -> Y1/1
  Data Type Conversion/1 -> Y7/1
  Data Type Conversion2/1 -> Y5/1

== system 8Bit_Processor/8-Bit_Processor/8-Bit 4-to-1 MUX/Subsystem ==
  I0 : Inport  OutDataTypeStr=boolean
  I1 : Inport  Port=2  OutDataTypeStr=boolean
  I2 : Inport  Port=3  OutDataTypeStr=boolean
  I3 : Inport  Port=4  OutDataTypeStr=boolean
  S : Inport  Port=5
  Logical Operator{,1..3} (4 alike) : Logic  Inputs=3  AllPortsSameDT=off  OutDataTypeStr=boolean
  Logical Operator4 : Logic  Operator=OR  Inputs=4  AllPortsSameDT=off  OutDataTypeStr=boolean
  NOT : Logic  Operator=NOT  IconShape=distinctive  AllPortsSameDT=off  OutDataTypeStr=boolean
  NOT1 : Logic  Operator=NOT  IconShape=distinctive  AllPortsSameDT=off  OutDataTypeStr=boolean
  Slicer : Subsystem
  Out1 : Outport  OutDataTypeStr=boolean
  wires:
  Logical Operator1/1 -> Logical Operator4/2
  NOT/1 -> Logical Operator/2, Logical Operator2/2
  I1/1 -> Logical Operator1/1
  I2/1 -> Logical Operator2/1
  NOT1/1 -> Logical Operator/3, Logical Operator1/3
  I3/1 -> Logical Operator3/1
  I0/1 -> Logical Operator/1
  Logical Operator2/1 -> Logical Operator4/3
  Logical Operator4/1 -> Out1/1
  Logical Operator3/1 -> Logical Operator4/4
  Logical Operator/1 -> Logical Operator4/1
  S/1 -> Slicer/1(X)
  Slicer/2(B) -> NOT1/1, Logical Operator2/3, Logical Operator3/3
  Slicer/1(A) -> NOT/1, Logical Operator1/2, Logical Operator3/2

== system 8Bit_Processor/8-Bit_Processor/8-Bit 4-to-1 MUX/Subsystem1 ==
  I0 : Inport  OutDataTypeStr=boolean
  I1 : Inport  Port=2  OutDataTypeStr=boolean
  I2 : Inport  Port=3  OutDataTypeStr=boolean
  I3 : Inport  Port=4  OutDataTypeStr=boolean
  S : Inport  Port=5
  Logical Operator{,1..3} (4 alike) : Logic  Inputs=3  AllPortsSameDT=off  OutDataTypeStr=boolean
  Logical Operator4 : Logic  Operator=OR  Inputs=4  AllPortsSameDT=off  OutDataTypeStr=boolean
  NOT : Logic  Operator=NOT  IconShape=distinctive  AllPortsSameDT=off  OutDataTypeStr=boolean
  NOT1 : Logic  Operator=NOT  IconShape=distinctive  AllPortsSameDT=off  OutDataTypeStr=boolean
  Slicer : Subsystem
  Out1 : Outport  OutDataTypeStr=boolean
  wires:
  Logical Operator1/1 -> Logical Operator4/2
  NOT/1 -> Logical Operator/2, Logical Operator2/2
  I1/1 -> Logical Operator1/1
  I2/1 -> Logical Operator2/1
  NOT1/1 -> Logical Operator/3, Logical Operator1/3
  I3/1 -> Logical Operator3/1
  I0/1 -> Logical Operator/1
  Logical Operator2/1 -> Logical Operator4/3
  Logical Operator4/1 -> Out1/1
  Logical Operator3/1 -> Logical Operator4/4
  Logical Operator/1 -> Logical Operator4/1
  S/1 -> Slicer/1(X)
  Slicer/2(B) -> NOT1/1, Logical Operator2/3, Logical Operator3/3
  Slicer/1(A) -> NOT/1, Logical Operator1/2, Logical Operator3/2

== system 8Bit_Processor/8-Bit_Processor/8-Bit 4-to-1 MUX/Subsystem2 ==
  I0 : Inport  OutDataTypeStr=boolean
  I1 : Inport  Port=2  OutDataTypeStr=boolean
  I2 : Inport  Port=3  OutDataTypeStr=boolean
  I3 : Inport  Port=4  OutDataTypeStr=boolean
  S : Inport  Port=5
  Logical Operator{,1..3} (4 alike) : Logic  Inputs=3  AllPortsSameDT=off  OutDataTypeStr=boolean
  Logical Operator4 : Logic  Operator=OR  Inputs=4  AllPortsSameDT=off  OutDataTypeStr=boolean
  NOT : Logic  Operator=NOT  IconShape=distinctive  AllPortsSameDT=off  OutDataTypeStr=boolean
  NOT1 : Logic  Operator=NOT  IconShape=distinctive  AllPortsSameDT=off  OutDataTypeStr=boolean
  Slicer : Subsystem
  Out1 : Outport  OutDataTypeStr=boolean
  wires:
  Logical Operator1/1 -> Logical Operator4/2
  NOT/1 -> Logical Operator/2, Logical Operator2/2
  I1/1 -> Logical Operator1/1
  I2/1 -> Logical Operator2/1
  NOT1/1 -> Logical Operator/3, Logical Operator1/3
  I3/1 -> Logical Operator3/1
  I0/1 -> Logical Operator/1
  Logical Operator2/1 -> Logical Operator4/3
  Logical Operator4/1 -> Out1/1
  Logical Operator3/1 -> Logical Operator4/4
  Logical Operator/1 -> Logical Operator4/1
  S/1 -> Slicer/1(X)
  Slicer/2(B) -> NOT1/1, Logical Operator2/3, Logical Operator3/3
  Slicer/1(A) -> NOT/1, Logical Operator1/2, Logical Operator3/2

== system 8Bit_Processor/8-Bit_Processor/8-Bit 4-to-1 MUX/Subsystem3 ==
  I0 : Inport  OutDataTypeStr=boolean
  I1 : Inport  Port=2  OutDataTypeStr=boolean
  I2 : Inport  Port=3  OutDataTypeStr=boolean
  I3 : Inport  Port=4  OutDataTypeStr=boolean
  S : Inport  Port=5
  Logical Operator{,1..3} (4 alike) : Logic  Inputs=3  AllPortsSameDT=off  OutDataTypeStr=boolean
  Logical Operator4 : Logic  Operator=OR  Inputs=4  AllPortsSameDT=off  OutDataTypeStr=boolean
  NOT : Logic  Operator=NOT  IconShape=distinctive  AllPortsSameDT=off  OutDataTypeStr=boolean
  NOT1 : Logic  Operator=NOT  IconShape=distinctive  AllPortsSameDT=off  OutDataTypeStr=boolean
  Slicer : Subsystem
  Out1 : Outport  OutDataTypeStr=boolean
  wires:
  Logical Operator1/1 -> Logical Operator4/2
  NOT/1 -> Logical Operator/2, Logical Operator2/2
  I1/1 -> Logical Operator1/1
  I2/1 -> Logical Operator2/1
  NOT1/1 -> Logical Operator/3, Logical Operator1/3
  I3/1 -> Logical Operator3/1
  I0/1 -> Logical Operator/1
  Logical Operator2/1 -> Logical Operator4/3
  Logical Operator4/1 -> Out1/1
  Logical Operator3/1 -> Logical Operator4/4
  Logical Operator/1 -> Logical Operator4/1
  S/1 -> Slicer/1(X)
  Slicer/2(B) -> NOT1/1, Logical Operator2/3, Logical Operator3/3
  Slicer/1(A) -> NOT/1, Logical Operator1/2, Logical Operator3/2

== system 8Bit_Processor/8-Bit_Processor/8-Bit 4-to-1 MUX/Subsystem4 ==
  I0 : Inport  OutDataTypeStr=boolean
  I1 : Inport  Port=2  OutDataTypeStr=boolean
  I2 : Inport  Port=3  OutDataTypeStr=boolean
  I3 : Inport  Port=4  OutDataTypeStr=boolean
  S : Inport  Port=5
  Logical Operator{,1..3} (4 alike) : Logic  Inputs=3  AllPortsSameDT=off  OutDataTypeStr=boolean
  Logical Operator4 : Logic  Operator=OR  Inputs=4  AllPortsSameDT=off  OutDataTypeStr=boolean
  NOT : Logic  Operator=NOT  IconShape=distinctive  AllPortsSameDT=off  OutDataTypeStr=boolean
  NOT1 : Logic  Operator=NOT  IconShape=distinctive  AllPortsSameDT=off  OutDataTypeStr=boolean
  Slicer : Subsystem
  Out1 : Outport  OutDataTypeStr=boolean
  wires:
  Logical Operator1/1 -> Logical Operator4/2
  NOT/1 -> Logical Operator/2, Logical Operator2/2
  I1/1 -> Logical Operator1/1
  I2/1 -> Logical Operator2/1
  NOT1/1 -> Logical Operator/3, Logical Operator1/3
  I3/1 -> Logical Operator3/1
  I0/1 -> Logical Operator/1
  Logical Operator2/1 -> Logical Operator4/3
  Logical Operator4/1 -> Out1/1
  Logical Operator3/1 -> Logical Operator4/4
  Logical Operator/1 -> Logical Operator4/1
  S/1 -> Slicer/1(X)
  Slicer/2(B) -> NOT1/1, Logical Operator2/3, Logical Operator3/3
  Slicer/1(A) -> NOT/1, Logical Operator1/2, Logical Operator3/2

== system 8Bit_Processor/8-Bit_Processor/8-Bit 4-to-1 MUX/Subsystem5 ==
  I0 : Inport  OutDataTypeStr=boolean
  I1 : Inport  Port=2  OutDataTypeStr=boolean
  I2 : Inport  Port=3  OutDataTypeStr=boolean
  I3 : Inport  Port=4  OutDataTypeStr=boolean
  S : Inport  Port=5
  Logical Operator{,1..3} (4 alike) : Logic  Inputs=3  AllPortsSameDT=off  OutDataTypeStr=boolean
  Logical Operator4 : Logic  Operator=OR  Inputs=4  AllPortsSameDT=off  OutDataTypeStr=boolean
  NOT : Logic  Operator=NOT  IconShape=distinctive  AllPortsSameDT=off  OutDataTypeStr=boolean
  NOT1 : Logic  Operator=NOT  IconShape=distinctive  AllPortsSameDT=off  OutDataTypeStr=boolean
  Slicer : Subsystem
  Out1 : Outport  OutDataTypeStr=boolean
  wires:
  Logical Operator1/1 -> Logical Operator4/2
  NOT/1 -> Logical Operator/2, Logical Operator2/2
  I1/1 -> Logical Operator1/1
  I2/1 -> Logical Operator2/1
  NOT1/1 -> Logical Operator/3, Logical Operator1/3
  I3/1 -> Logical Operator3/1
  I0/1 -> Logical Operator/1
  Logical Operator2/1 -> Logical Operator4/3
  Logical Operator4/1 -> Out1/1
  Logical Operator3/1 -> Logical Operator4/4
  Logical Operator/1 -> Logical Operator4/1
  S/1 -> Slicer/1(X)
  Slicer/2(B) -> NOT1/1, Logical Operator2/3, Logical Operator3/3
  Slicer/1(A) -> NOT/1, Logical Operator1/2, Logical Operator3/2

== system 8Bit_Processor/8-Bit_Processor/8-Bit 4-to-1 MUX/Subsystem6 ==
  I0 : Inport  OutDataTypeStr=boolean
  I1 : Inport  Port=2  OutDataTypeStr=boolean
  I2 : Inport  Port=3  OutDataTypeStr=boolean
  I3 : Inport  Port=4  OutDataTypeStr=boolean
  S : Inport  Port=5
  Logical Operator{,1..3} (4 alike) : Logic  Inputs=3  AllPortsSameDT=off  OutDataTypeStr=boolean
  Logical Operator4 : Logic  Operator=OR  Inputs=4  AllPortsSameDT=off  OutDataTypeStr=boolean
  NOT : Logic  Operator=NOT  IconShape=distinctive  AllPortsSameDT=off  OutDataTypeStr=boolean
  NOT1 : Logic  Operator=NOT  IconShape=distinctive  AllPortsSameDT=off  OutDataTypeStr=boolean
  Slicer : Subsystem
  Out1 : Outport  OutDataTypeStr=boolean
  wires:
  Logical Operator1/1 -> Logical Operator4/2
  NOT/1 -> Logical Operator/2, Logical Operator2/2
  I1/1 -> Logical Operator1/1
  I2/1 -> Logical Operator2/1
  NOT1/1 -> Logical Operator/3, Logical Operator1/3
  I3/1 -> Logical Operator3/1
  I0/1 -> Logical Operator/1
  Logical Operator2/1 -> Logical Operator4/3
  Logical Operator4/1 -> Out1/1
  Logical Operator3/1 -> Logical Operator4/4
  Logical Operator/1 -> Logical Operator4/1
  S/1 -> Slicer/1(X)
  Slicer/2(B) -> NOT1/1, Logical Operator2/3, Logical Operator3/3
  Slicer/1(A) -> NOT/1, Logical Operator1/2, Logical Operator3/2

== system 8Bit_Processor/8-Bit_Processor/8-Bit 4-to-1 MUX/Subsystem7 ==
  I0 : Inport  OutDataTypeStr=boolean
  I1 : Inport  Port=2  OutDataTypeStr=boolean
  I2 : Inport  Port=3  OutDataTypeStr=boolean
  I3 : Inport  Port=4  OutDataTypeStr=boolean
  S : Inport  Port=5
  Logical Operator{,1..3} (4 alike) : Logic  Inputs=3  AllPortsSameDT=off  OutDataTypeStr=boolean
  Logical Operator4 : Logic  Operator=OR  Inputs=4  AllPortsSameDT=off  OutDataTypeStr=boolean
  NOT : Logic  Operator=NOT  IconShape=distinctive  AllPortsSameDT=off  OutDataTypeStr=boolean
  NOT1 : Logic  Operator=NOT  IconShape=distinctive  AllPortsSameDT=off  OutDataTypeStr=boolean
  Slicer : Subsystem
  Out1 : Outport  OutDataTypeStr=boolean
  wires:
  Logical Operator1/1 -> Logical Operator4/2
  NOT/1 -> Logical Operator/2, Logical Operator2/2
  I1/1 -> Logical Operator1/1
  I2/1 -> Logical Operator2/1
  NOT1/1 -> Logical Operator/3, Logical Operator1/3
  I3/1 -> Logical Operator3/1
  I0/1 -> Logical Operator/1
  Logical Operator2/1 -> Logical Operator4/3
  Logical Operator4/1 -> Out1/1
  Logical Operator3/1 -> Logical Operator4/4
  Logical Operator/1 -> Logical Operator4/1
  S/1 -> Slicer/1(X)
  Slicer/2(B) -> NOT1/1, Logical Operator2/3, Logical Operator3/3
  Slicer/1(A) -> NOT/1, Logical Operator1/2, Logical Operator3/2

== system 8Bit_Processor/8-Bit_Processor/8-Bit_Adder/Concat1 ==
  X7 : Inport  OutDataTypeStr=boolean  SampleTime=1
  X6 : Inport  Port=2  OutDataTypeStr=boolean  SampleTime=1
  X5 : Inport  Port=3  OutDataTypeStr=boolean  SampleTime=1
  X4 : Inport  Port=4  OutDataTypeStr=boolean  SampleTime=1
  X3 : Inport  Port=5  OutDataTypeStr=boolean  SampleTime=1
  X2 : Inport  Port=6  OutDataTypeStr=boolean  SampleTime=1
  X1 : Inport  Port=7  OutDataTypeStr=boolean  SampleTime=1
  X0 : Inport  Port=8  OutDataTypeStr=boolean  SampleTime=1
  Bit Concat : hdlsllib/Logic and Bit Operations/Bit Concat  numInputs=8
      settings: SourceProductName=Simulink
  Y : Outport
  wires:
  X6/1 -> Bit Concat/2
  X2/1 -> Bit Concat/6
  X7/1 -> Bit Concat/1
  X0/1 -> Bit Concat/8
  Bit Concat/1 -> Y/1
  X3/1 -> Bit Concat/5
  X1/1 -> Bit Concat/7
  X5/1 -> Bit Concat/3
  X4/1 -> Bit Concat/4

== system 8Bit_Processor/8-Bit_Processor/8-Bit_Adder/Full adder1 ==
  In1 : Inport  OutDataTypeStr=boolean
  In2 : Inport  Port=2  OutDataTypeStr=boolean
  In3 : Inport  Port=3  OutDataTypeStr=boolean
  Half adder1 : Subsystem
  Half adder2 : Subsystem
  Logical Operator1 : Logic  Operator=OR  AllPortsSameDT=off  OutDataTypeStr=boolean
  Out1 : Outport
  Out2 : Outport  Port=2
  wires:
  Logical Operator1/1 -> Out2/1
  In1/1 -> Half adder1/1(In1)
  Half adder2/1(Out1) -> Out1/1
  In2/1 -> Half adder1/2(In2)
  In3/1 -> Half adder2/2(In2)
  Half adder1/2(Out2) -> Logical Operator1/2
  Half adder1/1(Out1) -> Half adder2/1(In1)
  Half adder2/2(Out2) -> Logical Operator1/1

== system 8Bit_Processor/8-Bit_Processor/8-Bit_Adder/Full adder2 ==
  In1 : Inport  OutDataTypeStr=boolean
  In2 : Inport  Port=2  OutDataTypeStr=boolean
  In3 : Inport  Port=3  OutDataTypeStr=boolean
  Half adder1 : Subsystem
  Half adder2 : Subsystem
  Logical Operator1 : Logic  Operator=OR  AllPortsSameDT=off  OutDataTypeStr=boolean
  Out1 : Outport
  Out2 : Outport  Port=2
  wires:
  Logical Operator1/1 -> Out2/1
  In1/1 -> Half adder1/1(In1)
  Half adder2/1(Out1) -> Out1/1
  In2/1 -> Half adder1/2(In2)
  In3/1 -> Half adder2/2(In2)
  Half adder1/2(Out2) -> Logical Operator1/2
  Half adder1/1(Out1) -> Half adder2/1(In1)
  Half adder2/2(Out2) -> Logical Operator1/1

== system 8Bit_Processor/8-Bit_Processor/8-Bit_Adder/Full adder3 ==
  In1 : Inport  OutDataTypeStr=boolean
  In2 : Inport  Port=2  OutDataTypeStr=boolean
  In3 : Inport  Port=3  OutDataTypeStr=boolean
  Half adder1 : Subsystem
  Half adder2 : Subsystem
  Logical Operator1 : Logic  Operator=OR  AllPortsSameDT=off  OutDataTypeStr=boolean
  Out1 : Outport
  Out2 : Outport  Port=2
  wires:
  Logical Operator1/1 -> Out2/1
  In1/1 -> Half adder1/1(In1)
  Half adder2/1(Out1) -> Out1/1
  In2/1 -> Half adder1/2(In2)
  In3/1 -> Half adder2/2(In2)
  Half adder1/2(Out2) -> Logical Operator1/2
  Half adder1/1(Out1) -> Half adder2/1(In1)
  Half adder2/2(Out2) -> Logical Operator1/1

== system 8Bit_Processor/8-Bit_Processor/8-Bit_Adder/Full adder4 ==
  In1 : Inport  OutDataTypeStr=boolean
  In2 : Inport  Port=2  OutDataTypeStr=boolean
  In3 : Inport  Port=3  OutDataTypeStr=boolean
  Half adder1 : Subsystem
  Half adder2 : Subsystem
  Logical Operator1 : Logic  Operator=OR  AllPortsSameDT=off  OutDataTypeStr=boolean
  Out1 : Outport
  Out2 : Outport  Port=2
  wires:
  Logical Operator1/1 -> Out2/1
  In1/1 -> Half adder1/1(In1)
  Half adder2/1(Out1) -> Out1/1
  In2/1 -> Half adder1/2(In2)
  In3/1 -> Half adder2/2(In2)
  Half adder1/2(Out2) -> Logical Operator1/2
  Half adder1/1(Out1) -> Half adder2/1(In1)
  Half adder2/2(Out2) -> Logical Operator1/1

== system 8Bit_Processor/8-Bit_Processor/8-Bit_Adder/Full adder5 ==
  In1 : Inport  OutDataTypeStr=boolean
  In2 : Inport  Port=2  OutDataTypeStr=boolean
  In3 : Inport  Port=3  OutDataTypeStr=boolean
  Half adder1 : Subsystem
  Half adder2 : Subsystem
  Logical Operator1 : Logic  Operator=OR  AllPortsSameDT=off  OutDataTypeStr=boolean
  Out1 : Outport
  Out2 : Outport  Port=2
  wires:
  Logical Operator1/1 -> Out2/1
  In1/1 -> Half adder1/1(In1)
  Half adder2/1(Out1) -> Out1/1
  In2/1 -> Half adder1/2(In2)
  In3/1 -> Half adder2/2(In2)
  Half adder1/2(Out2) -> Logical Operator1/2
  Half adder1/1(Out1) -> Half adder2/1(In1)
  Half adder2/2(Out2) -> Logical Operator1/1

== system 8Bit_Processor/8-Bit_Processor/8-Bit_Adder/Full adder6 ==
  In1 : Inport  OutDataTypeStr=boolean
  In2 : Inport  Port=2  OutDataTypeStr=boolean
  In3 : Inport  Port=3  OutDataTypeStr=boolean
  Half adder1 : Subsystem
  Half adder2 : Subsystem
  Logical Operator1 : Logic  Operator=OR  AllPortsSameDT=off  OutDataTypeStr=boolean
  Out1 : Outport
  Out2 : Outport  Port=2
  wires:
  Logical Operator1/1 -> Out2/1
  In1/1 -> Half adder1/1(In1)
  Half adder2/1(Out1) -> Out1/1
  In2/1 -> Half adder1/2(In2)
  In3/1 -> Half adder2/2(In2)
  Half adder1/2(Out2) -> Logical Operator1/2
  Half adder1/1(Out1) -> Half adder2/1(In1)
  Half adder2/2(Out2) -> Logical Operator1/1

== system 8Bit_Processor/8-Bit_Processor/8-Bit_Adder/Full adder7 ==
  In1 : Inport  OutDataTypeStr=boolean
  In2 : Inport  Port=2  OutDataTypeStr=boolean
  In3 : Inport  Port=3  OutDataTypeStr=boolean
  Half adder1 : Subsystem
  Half adder2 : Subsystem
  Logical Operator1 : Logic  Operator=OR  AllPortsSameDT=off  OutDataTypeStr=boolean
  Out1 : Outport
  Out2 : Outport  Port=2
  wires:
  Logical Operator1/1 -> Out2/1
  In1/1 -> Half adder1/1(In1)
  Half adder2/1(Out1) -> Out1/1
  In2/1 -> Half adder1/2(In2)
  In3/1 -> Half adder2/2(In2)
  Half adder1/2(Out2) -> Logical Operator1/2
  Half adder1/1(Out1) -> Half adder2/1(In1)
  Half adder2/2(Out2) -> Logical Operator1/1

== system 8Bit_Processor/8-Bit_Processor/8-Bit_Adder/Half adder1 ==
  In1 : Inport  OutDataTypeStr=boolean
  In2 : Inport  Port=2  OutDataTypeStr=boolean
  Logical Operator : Logic  AllPortsSameDT=off  OutDataTypeStr=boolean
  Logical Operator1 : Logic  Operator=XOR  AllPortsSameDT=off  OutDataTypeStr=boolean
  Out1 : Outport
  Out2 : Outport  Port=2
  wires:
  In2/1 -> Logical Operator/2, Logical Operator1/2
  In1/1 -> Logical Operator/1, Logical Operator1/1
  Logical Operator1/1 -> Out1/1
  Logical Operator/1 -> Out2/1
